simulink model "step6"  (Simulink 10.2)
settings: Solver=FixedStepAuto  StartTime=0.0  StopTime=3  FixedStep=T_step  RelTol=1e-3
values from neighbouring files (symbols this model uses):
  F = [Fx;Fy;Mz]    [Jacobi_T.m]    (also in PRBDM_CTC_task.m = M_tilda*v+C_tilda*dX+G_tilda; RRR_CTC_task.m = M_tilda*v+V_tilda*dX+G_tilda; RRR_jtraj.m = q0; step2.mat = 10)
  gama0 = Rparams4dyn(3)    [PRBDM_3R_Dynamic_Matrices_Lagrange.m]    (also in PRBDM_3R_Dynamics.m = in4dyn(12); PRBDM_3R_Dynamics00.m = in4dyn(12); PRBDM_3R_DynamicsPID.m = in4dyn(12); PRBDM_3R_parameters.m = 0.1)
  gama1 = x(7)    [Jacobi_T.m]    (also in PRBDM_3R_Dynamic_Matrices_Lagrange.m = Rparams4dyn(4); PRBDM_3R_Dynamics.m = in4dyn(13); PRBDM_3R_Dynamics00.m = in4dyn(13); PRBDM_3R_DynamicsPID.m = in4dyn(13))
  gama2 = x(8)    [Jacobi_T.m]    (also in PRBDM_3R_Dynamic_Matrices_Lagrange.m = Rparams4dyn(5); PRBDM_3R_Dynamics.m = in4dyn(14); PRBDM_3R_Dynamics00.m = in4dyn(14); PRBDM_3R_DynamicsPID.m = in4dyn(14))
  gama3 = x(9)    [Jacobi_T.m]    (also in PRBDM_3R_Dynamic_Matrices_Lagrange.m = Rparams4dyn(6); PRBDM_3R_Dynamics.m = in4dyn(15); PRBDM_3R_Dynamics00.m = in4dyn(15); PRBDM_3R_DynamicsPID.m = in4dyn(15))
  I = Rparams4dyn(10)    [PRBDM_3R_Dynamic_Matrices_Lagrange.m]    (also in PRBDM_3R_Dynamics.m = in4dyn(19); PRBDM_3R_Dynamics00.m = in4dyn(19); PRBDM_3R_DynamicsPID.m = in4dyn(19); PRBDM_3R_parameters.m = 1.8e-11)
  k1 = Rparams4dyn(7)    [PRBDM_3R_Dynamic_Matrices_Lagrange.m]    (also in PRBDM_3R_Dynamics.m = in4dyn(16); PRBDM_3R_Dynamics00.m = in4dyn(16); PRBDM_3R_DynamicsPID.m = in4dyn(16); PRBDM_3R_parameters.m = 0.290628)
  k2 = Rparams4dyn(8)    [PRBDM_3R_Dynamic_Matrices_Lagrange.m]    (also in PRBDM_3R_Dynamics.m = in4dyn(17); PRBDM_3R_Dynamics00.m = in4dyn(17); PRBDM_3R_DynamicsPID.m = in4dyn(17); PRBDM_3R_parameters.m = 0.247572)
  k3 = Rparams4dyn(9)    [PRBDM_3R_Dynamic_Matrices_Lagrange.m]    (also in PRBDM_3R_Dynamics.m = in4dyn(18); PRBDM_3R_Dynamics00.m = in4dyn(18); PRBDM_3R_DynamicsPID.m = in4dyn(18); PRBDM_3R_parameters.m = 0.213624)
  L = Rparams4dyn(2)    [PRBDM_3R_Dynamic_Matrices_Lagrange.m]    (also in PRBDM_3R_Dynamics.m = in4dyn(11); PRBDM_3R_Dynamics00.m = in4dyn(11); PRBDM_3R_DynamicsPID.m = in4dyn(11); PRBDM_3R_parameters.m = 0.3)
  L0 = z(7)    [Forward_kinematics.m]    (also in GeometricCalculation_simulink.m = Geoparams(4); PRBDM_3R_parameters.m = 0.03; PRBDM_3R_parameters.mat = 0.03; TrajectoryPlanning_simulink.m = X(8))
  L1 = z(8)    [Forward_kinematics.m]    (also in GeometricCalculation_simulink.m = Geoparams(5); Jacobi.m = x(4); PRBDM_3R_CTC.m = x(19); PRBDM_3R_Dynamic_Matrices_NewtonEular.m = robot_params(4))
  L2 = z(9)    [Forward_kinematics.m]    (also in GeometricCalculation_simulink.m = Geoparams(6); Jacobi.m = x(5); PRBDM_3R_CTC.m = x(20); PRBDM_3R_Dynamic_Matrices_NewtonEular.m = robot_params(5))
  L3 = z(10)    [Forward_kinematics.m]    (also in GeometricCalculation_simulink.m = Geoparams(7); Jacobi.m = x(6); PRBDM_3R_CTC.m = x(21); PRBDM_3R_Dynamic_Matrices_NewtonEular.m = robot_params(6))
  m = Rparams4dyn(1)    [PRBDM_3R_Dynamic_Matrices_Lagrange.m]    (also in PRBDM_3R_Dynamics.m = in4dyn(10); PRBDM_3R_Dynamics00.m = in4dyn(10); PRBDM_3R_DynamicsPID.m = in4dyn(10); PRBDM_3R_parameters.m = 1)
  Mz = x(6)    [Jacobi_T.m]    (also in step2.mat = 10; step2_trajectory.m = 10; step3.m = 10)
  phi_f = 1.0471975512    [step2.mat]    (also in step2_trajectory.m; step3.m)
  W = x(22)    [PRBDM_3R_CTC.m]    (also in PRBDM_3R_Dynamic_Matrices_NewtonEular.m = robot_params(7); PRBDM_3R_Dynamics.m = in4dyn(20); PRBDM_3R_Dynamics00.m = in4dyn(20); PRBDM_3R_DynamicsPID.m = in4dyn(20))
  x_f = 0.0536    [step2.mat]    (also in step2_trajectory.m; step3.m)
  y_f = 0.135    [step2.mat]    (also in step2_trajectory.m; step3.m)
settings Model: Creator=Master  LastModifiedBy=Master
settings DataIOCC: SaveFormat=Dataset  SignalLoggingSaveFormat=Dataset  ReturnWorkspaceOutputs=on
settings OptimizationCC: LifeSpan=auto
settings DebuggingCC: UnderspecifiedInitializationDetection=Simplified  MergeDetectMultiDrivingBlocksExec=error  FcnCallInpInsideContextMsg=error  SFUnexpectedBacktrackingDiag=error  SFNoUnconditionalDefaultTransitionDiag=error  SFExecutionAtInitializationDiag=warning  ArithmeticOperatorsInVariantConditions=error
settings HardwareCC: ProdBitPerPointer=64  ProdBitPerSizeT=64  ProdBitPerPtrDiffT=64  ProdLargestAtomicFloat=Float  ProdIntDivRoundTo=Zero  ProdEndianess=LittleEndian  ProdWordSize=64  ProdHWDeviceType=Intel->x86-64 (Windows64)
settings ModelReferenceCC: PropagateSignalLabelsOutOfModel=on
settings SFSimCC: SimUseLocalCustomCode=on  CustomCodeUndefinedFunction=FilterOut
settings RTWCC: RTWUseLocalCustomCode=on
settings CodeAppCC: StateflowObjectComments=off
settings GRTTargetCC: TargetLangStandard=C99 (ISO)  CombineOutputUpdateFcns=on  GRTInterface=off
settings ConfigComp: CovMetricSettings=dwe  CovSaveCumulativeToWorkspaceVar=off  CovSaveSingleToWorkspaceVar=off  CovExternalEMLEnable=on

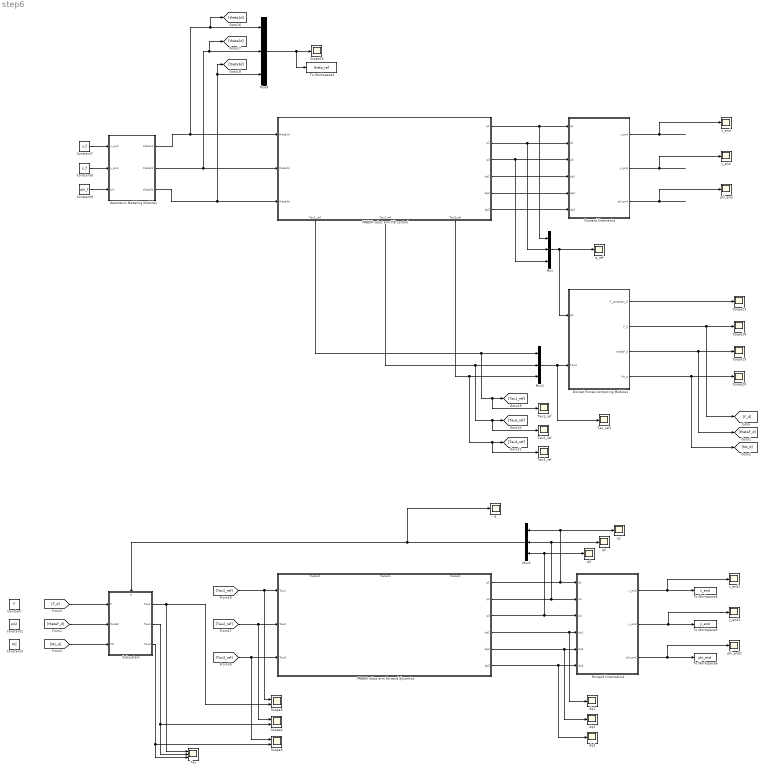
== system step6 ==
  Constant : Constant  Value=F
  Constant1 : Constant  Value=pi/2
  Constant3 : Constant  Value=Mz
  Constant7 : Constant  Value=x_f
  Constant8 : Constant  Value=y_f
  Constant9 : Constant  Value=phi_f
  Disired Forces Computing Module1 : Subsystem
  Forward kinematics : Subsystem
  Forward kinematics1 : Subsystem
  Geometric Modeling Module1 : Subsystem
  Mux{,1..2,9} (4 alike) : Mux  Inputs=3
  PRBDM robot arm Forward dynamics : Subsystem
      settings: PortSchema="{\"entries\":[{\"content\":{\"sides\":[{\"content\":{\"connectorIds\":[\"In1\",\"In2\",\"In3\"]},\"type\":\"ConnectorPlacement.EquallySpacedRectSide\",\"uuid\":\"1f88892b-0bd0-49de-aca9-2c32e7693572\"},{\"content\":{\"connectorIds\":[\"Out1\",\"Out2\",\"Out3\",\"Out4\",\"Out5\",\"Out6\"],\"side\":\"RIGHT\"},\"type\":\"ConnectorPlacement.EquallySpacedRectSide\",\"uuid\":\"b703a21d-fa56-4217-8064-1c2098ab3c38\"},{\"content\":{\"connectorIds\":[\"In4\",\"In5\",\"In6\"],\"side\":\"TOP\"},\"type\":\"ConnectorPlacement.EquallySpacedRectSide\",\"uuid\":\"2526ef97-18a1-4ac3-963d-0ba7d1a2d319\"},{\"content\":{\"connectorIds\":[],\"side\":\"BOTTOM\"},\"type\":\"ConnectorPlacement.EquallySpacedRectSide\",\"uuid\":\"f33fbcfd-8e0b-408f-a669-776188a4cff3\"},{\"content\":{\"connectorIds\":[],\"side\":\"HIDDEN\"},\"type\":\"ConnectorPlacement.EquallySpacedRectSide\",\"uuid\":\"8c9044ff-40c0-4995-b32e-bf50be4b71db\"}]},\"type\":\"ConnectorPlacement.EquallySpacedConnector\",\"uuid\":\"32b5ad01-d59a-45fa-aad8-e0a4c9d304fb\"}],\"packageUris\":[\"http://schema.mathworks.com/mf0/Connector/R2020b\"],\"version\":\"1.0\"}"
      mask Display: image(imread('RRR.png'))
  PRBDM robot arm PID control : Subsystem
      settings: PortSchema="{\"entries\":[{\"content\":{\"sides\":[{\"content\":{\"connectorIds\":[\"In1\",\"In2\",\"In3\"]},\"type\":\"ConnectorPlacement.EquallySpacedRectSide\",\"uuid\":\"1f88892b-0bd0-49de-aca9-2c32e7693572\"},{\"content\":{\"connectorIds\":[\"Out1\",\"Out2\",\"Out3\",\"Out4\",\"Out5\",\"Out6\"],\"side\":\"RIGHT\"},\"type\":\"ConnectorPlacement.EquallySpacedRectSide\",\"uuid\":\"b703a21d-fa56-4217-8064-1c2098ab3c38\"},{\"content\":{\"connectorIds\":[],\"side\":\"TOP\"},\"type\":\"ConnectorPlacement.EquallySpacedRectSide\",\"uuid\":\"2526ef97-18a1-4ac3-963d-0ba7d1a2d319\"},{\"content\":{\"connectorIds\":[\"Out7\",\"Out8\",\"Out9\"],\"side\":\"BOTTOM\"},\"type\":\"ConnectorPlacement.EquallySpacedRectSide\",\"uuid\":\"f33fbcfd-8e0b-408f-a669-776188a4cff3\"},{\"content\":{\"connectorIds\":[],\"side\":\"HIDDEN\"},\"type\":\"ConnectorPlacement.EquallySpacedRectSide\",\"uuid\":\"8c9044ff-40c0-4995-b32e-bf50be4b71db\"}]},\"type\":\"ConnectorPlacement.EquallySpacedConnector\",\"uuid\":\"32b5ad01-d59a-45fa-aad8-e0a4c9d304fb\"}],\"packageUris\":[\"http://schema.mathworks.com/mf0/Connector/R2020b\"],\"version\":\"1.0\"}"
      mask Display: image(imread('RRR.png'))
  Scope{16,18..20,23} (5 alike) : Scope
  Scope2 : Scope  NumInputPorts=2
  Scope3 : Scope  NumInputPorts=2
  Scope5 : Scope  NumInputPorts=2
  Subsystem : Subsystem
      settings: PortSchema="{\"entries\":[{\"content\":{\"sides\":[{\"content\":{\"connectorIds\":[\"In1\",\"In2\",\"In3\"]},\"type\":\"ConnectorPlacement.EquallySpacedRectSide\",\"uuid\":\"03e3fa68-98df-40a7-88fb-f274e89646de\"},{\"content\":{\"connectorIds\":[\"Out1\",\"Out2\",\"Out3\"],\"side\":\"RIGHT\"},\"type\":\"ConnectorPlacement.EquallySpacedRectSide\",\"uuid\":\"1a7c6e69-d785-4f03-b0d8-74a38f8f42a1\"},{\"content\":{\"connectorIds\":[\"In4\"],\"side\":\"TOP\"},\"type\":\"ConnectorPlacement.EquallySpacedRectSide\",\"uuid\":\"61c135cb-8cc5-493d-9c37-8230cda997e1\"},{\"content\":{\"connectorIds\":[],\"side\":\"HIDDEN\"},\"type\":\"ConnectorPlacement.EquallySpacedRectSide\",\"uuid\":\"5d99950e-feb6-474c-993a-cad470b06503\"}]},\"type\":\"ConnectorPlacement.EquallySpacedConnector\",\"uuid\":\"5533c5e9-db4a-4e3a-8115-8d67f8979e0c\"}],\"packageUris\":[\"http://schema.mathworks.com/mf0/Connector/R2020b\"],\"version\":\"1.0\"}"
  Tau : Scope  NumInputPorts=3
  Tau1_ref : Scope
  Tau2_ref : Scope
  Tau3_ref : Scope
  Tau_ref1 : Scope
  To Workspace3 : ToWorkspace  VariableName=theta_ref  SaveFormat=Timeseries  SampleTime=-1
  To Workspace4 : ToWorkspace  VariableName=x_end  SampleTime=-1
  To Workspace5 : ToWorkspace  VariableName=y_end  SampleTime=-1
  To Workspace6 : ToWorkspace  VariableName=phi_end  SampleTime=-1
  dq1 : Scope
  dq2 : Scope
  dq3 : Scope
  phi_end : Scope
  phi_end1 : Scope
  q{,1..3} (4 alike) : Scope
  q_ref : Scope
  x_end : Scope
  x_end1 : Scope
  y_end : Scope
  y_end1 : Scope
  wires:
  Mux9/1 -> To Workspace3/1, Scope16/1
  Geometric Modeling Module1/3(theta3d) -> [theta3d], Mux9/3, PRBDM robot arm PID control/3(theta3d)
  Constant9/1 -> Geometric Modeling Module1/3(phi)
  Constant7/1 -> Geometric Modeling Module1/1(x_end)
  Constant8/1 -> Geometric Modeling Module1/2(y_end)
  Geometric Modeling Module1/1(theta1d) -> PRBDM robot arm PID control/1(theta1d), [theta1d], Mux9/1
  Geometric Modeling Module1/2(theta2d) -> PRBDM robot arm PID control/2(theta2d), [theta2d], Mux9/2
  Mux/1 -> q_ref/1, Disired Forces Computing Module1/1(qd)
  PRBDM robot arm PID control/5(dq2) -> Forward kinematics/5(dq2)
  PRBDM robot arm PID control/1(q1) -> Mux/1, Forward kinematics/1(q1)
  PRBDM robot arm PID control/6(dq3) -> Forward kinematics/6(dq3)
  PRBDM robot arm PID control/4(dq1) -> Forward kinematics/4(dq1)
  Forward kinematics/1(x_end) -> x_end/1
  PRBDM robot arm PID control/2(q2) -> Forward kinematics/2(q2), Mux/2
  Forward kinematics/3(phi_end) -> phi_end/1
  Forward kinematics/2(y_end) -> y_end/1
  PRBDM robot arm PID control/3(q3) -> Forward kinematics/3(q3), Mux/3
  Disired Forces Computing Module1/4(Mz_d) -> [Mz_d], Scope20/1
  Disired Forces Computing Module1/3(thetaF_d) -> [thetaF_d], Scope19/1
  Disired Forces Computing Module1/2(F_d) -> [F_d], Scope18/1
  Disired Forces Computing Module1/1(F_cartesian_d) -> Scope23/1
  PRBDM robot arm PID control/8(Tau2_ref) -> Tau2_ref/1, [Tau2_ref], Mux1/2
  PRBDM robot arm PID control/7(Tau1_ref) -> Tau1_ref/1, [Tau1_ref], Mux1/1
  Mux1/1 -> Tau_ref1/1, Disired Forces Computing Module1/2(Taud)
  PRBDM robot arm PID control/9(Tau3_ref) -> Tau3_ref/1, [Tau3_ref], Mux1/3
  Forward kinematics1/2(y_end) -> y_end1/1, To Workspace5/1
  PRBDM robot arm Forward dynamics/2(q2) -> q2/1, Mux2/2, Forward kinematics1/2(q2)
  PRBDM robot arm Forward dynamics/3(q3) -> q3/1, Mux2/3, Forward kinematics1/3(q3)
  Forward kinematics1/1(x_end) -> To Workspace4/1, x_end1/1
  PRBDM robot arm Forward dynamics/4(dq1) -> dq1/1, Forward kinematics1/4(dq1)
  PRBDM robot arm Forward dynamics/6(dq3) -> dq3/1, Forward kinematics1/6(dq3)
  PRBDM robot arm Forward dynamics/5(dq2) -> dq2/1, Forward kinematics1/5(dq2)
  PRBDM robot arm Forward dynamics/1(q1) -> Mux2/1, q1/1, Forward kinematics1/1(q1)
  Mux2/1 -> Subsystem/4(q), q/1
  Forward kinematics1/3(phi_end) -> phi_end1/1, To Workspace6/1
  [Mz_d] -> Subsystem/3(Mz)
  [thetaF_d] -> Subsystem/2(thetaF)
  [F_d] -> Subsystem/1(F)
  [Tau1_ref] -> Scope5/1, PRBDM robot arm Forward dynamics/1(Tau1)
  [Tau2_ref] -> Scope2/1, PRBDM robot arm Forward dynamics/2(Tau2)
  [Tau3_ref] -> Scope3/1, PRBDM robot arm Forward dynamics/3(Tau3)
  Subsystem/1(Tau1) -> Tau/1, Scope5/2
  Subsystem/2(Tau2) -> Scope2/2, Tau/2
  Subsystem/3(Tau3) -> Scope3/2, Tau/3

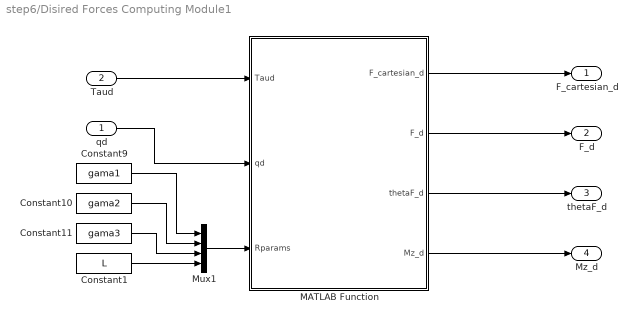
== system step6/Disired Forces Computing Module1 ==
  qd : Inport
  Taud : Inport  Port=2
  Constant1 : Constant  Value=L
  Constant10 : Constant  Value=gama2
  Constant11 : Constant  Value=gama3
  Constant9 : Constant  Value=gama1
  MATLAB Function : MATLAB Function  TreatAsAtomicUnit=on
  Mux1 : Mux
  F_cartesian_d : Outport
  F_d : Outport  Port=2
  thetaF_d : Outport  Port=3
  Mz_d : Outport  Port=4
  wires:
  MATLAB Function/1(F_cartesian_d) -> F_cartesian_d/1
  Mux1/1 -> MATLAB Function/3(Rparams)
  Constant9/1 -> Mux1/1
  Constant10/1 -> Mux1/2
  Constant11/1 -> Mux1/3
  Taud/1 -> MATLAB Function/1(Taud)
  qd/1 -> MATLAB Function/2(qd)
  Constant1/1 -> Mux1/4
  MATLAB Function/2(F_d) -> F_d/1
  MATLAB Function/3(thetaF_d) -> thetaF_d/1
  MATLAB Function/4(Mz_d) -> Mz_d/1

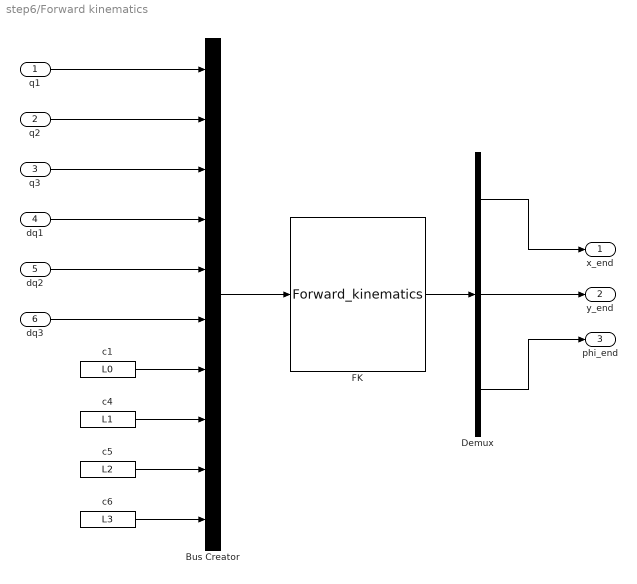
== system step6/Forward kinematics ==
  q1 : Inport
  q2 : Inport  Port=2
  q3 : Inport  Port=3
  dq1 : Inport  Port=4
  dq2 : Inport  Port=5
  dq3 : Inport  Port=6
  Bus Creator : BusCreator  Inputs=10
  Demux : Demux  Outputs=3
  FK : MATLABFcn  MATLABFcn=Forward_kinematics  OutputDimensions=3
  c1 : Constant  Value=L0
  c4 : Constant  Value=L1
  c5 : Constant  Value=L2
  c6 : Constant  Value=L3
  x_end : Outport
  y_end : Outport  Port=2
  phi_end : Outport  Port=3
  wires:
  c6/1 -> Bus Creator/10
  Demux/1 -> x_end/1
  c4/1 -> Bus Creator/8
  q2/1 -> Bus Creator/2
  q1/1 -> Bus Creator/1
  q3/1 -> Bus Creator/3
  Bus Creator/1 -> FK/1
  dq2/1 -> Bus Creator/5
  Demux/2 -> y_end/1
  FK/1 -> Demux/1
  dq1/1 -> Bus Creator/4
  Demux/3 -> phi_end/1
  dq3/1 -> Bus Creator/6
  c5/1 -> Bus Creator/9
  c1/1 -> Bus Creator/7

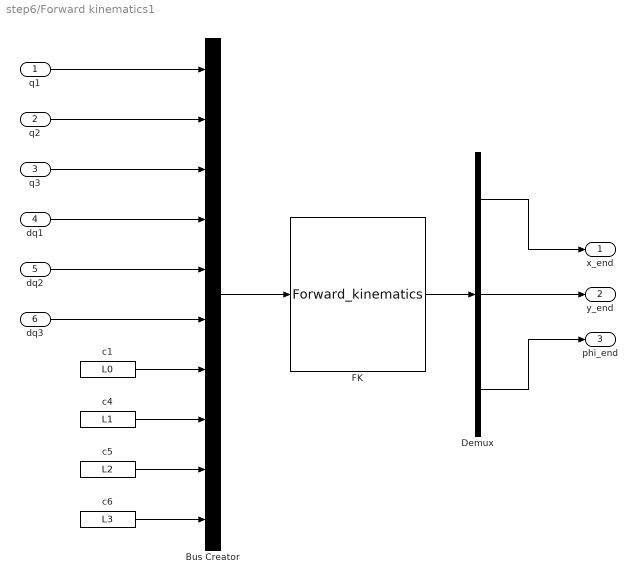
== system step6/Forward kinematics1 ==
  q1 : Inport
  q2 : Inport  Port=2
  q3 : Inport  Port=3
  dq1 : Inport  Port=4
  dq2 : Inport  Port=5
  dq3 : Inport  Port=6
  Bus Creator : BusCreator  Inputs=10
  Demux : Demux  Outputs=3
  FK : MATLABFcn  MATLABFcn=Forward_kinematics  OutputDimensions=3
  c1 : Constant  Value=L0
  c4 : Constant  Value=L1
  c5 : Constant  Value=L2
  c6 : Constant  Value=L3
  x_end : Outport
  y_end : Outport  Port=2
  phi_end : Outport  Port=3
  wires:
  c6/1 -> Bus Creator/10
  Demux/1 -> x_end/1
  c4/1 -> Bus Creator/8
  q2/1 -> Bus Creator/2
  q1/1 -> Bus Creator/1
  q3/1 -> Bus Creator/3
  Bus Creator/1 -> FK/1
  dq2/1 -> Bus Creator/5
  Demux/2 -> y_end/1
  FK/1 -> Demux/1
  dq1/1 -> Bus Creator/4
  Demux/3 -> phi_end/1
  dq3/1 -> Bus Creator/6
  c5/1 -> Bus Creator/9
  c1/1 -> Bus Creator/7

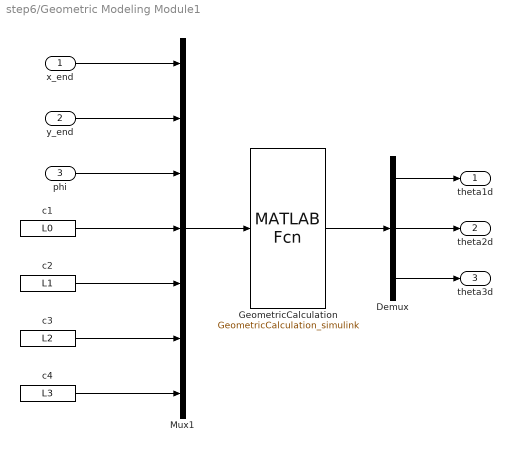
== system step6/Geometric Modeling Module1 ==
  x_end : Inport
  y_end : Inport  Port=2
  phi : Inport  Port=3
  Demux : Demux  Outputs=3
  GeometricCalculation : MATLABFcn  MATLABFcn=GeometricCalculation_simulink
  Mux1 : Mux  Inputs=7
  c1 : Constant  Value=L0
  c2 : Constant  Value=L1
  c3 : Constant  Value=L2
  c4 : Constant  Value=L3
  theta1d : Outport
  theta2d : Outport  Port=2
  theta3d : Outport  Port=3
  wires:
  Mux1/1 -> GeometricCalculation/1
  y_end/1 -> Mux1/2
  x_end/1 -> Mux1/1
  phi/1 -> Mux1/3
  c1/1 -> Mux1/4
  c3/1 -> Mux1/6
  c2/1 -> Mux1/5
  GeometricCalculation/1 -> Demux/1
  Demux/2 -> theta2d/1
  Demux/1 -> theta1d/1
  Demux/3 -> theta3d/1
  c4/1 -> Mux1/7

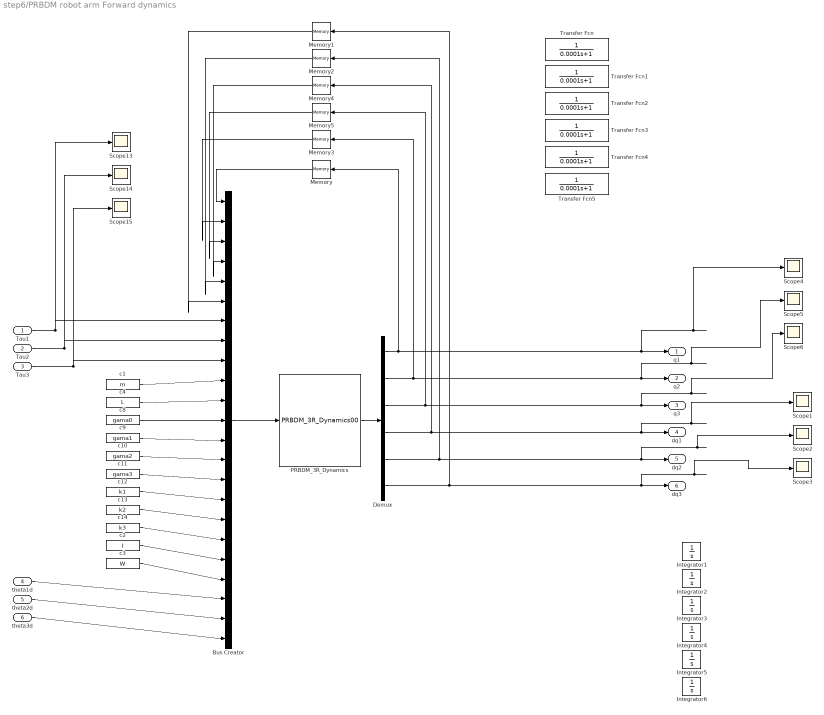
== system step6/PRBDM robot arm Forward dynamics ==
  Tau1 : Inport
  Tau2 : Inport  Port=2
  Tau3 : Inport  Port=3
  theta1d : Inport  Port=4
  theta2d : Inport  Port=5
  theta3d : Inport  Port=6
  Bus Creator : BusCreator  Inputs=23
  Demux : Demux  Outputs=6
  Integrator{1..6} (6 alike) : Integrator  UpperSaturationLimit=1e6  LowerSaturationLimit=-1e6
  Memory{,1..5} (6 alike) : Memory
  PRBDM_3R_Dynamics : MATLABFcn  MATLABFcn=PRBDM_3R_Dynamics00  OutputDimensions=6
  Scope{1..6,13..15} (9 alike) : Scope
  Transfer Fcn{,1..5} (6 alike) : TransferFcn  Denominator=[0.0001 1]
  c1 : Constant  Value=m
  c10 : Constant  Value=gama2
  c11 : Constant  Value=gama3
  c12 : Constant  Value=k1
  c13 : Constant  Value=k2
  c14 : Constant  Value=k3
  c2 : Constant  Value=I
  c3 : Constant  Value=W
  c4 : Constant  Value=L
  c8 : Constant  Value=gama0
  c9 : Constant  Value=gama1
  q1 : Outport
  q2 : Outport  Port=2
  q3 : Outport  Port=3
  dq1 : Outport  Port=4
  dq2 : Outport  Port=5
  dq3 : Outport  Port=6
  wires:
  theta3d/1 -> Bus Creator/23
  theta2d/1 -> Bus Creator/22
  c11/1 -> Bus Creator/15
  c3/1 -> Bus Creator/20
  c14/1 -> Bus Creator/18
  c2/1 -> Bus Creator/19
  c1/1 -> Bus Creator/10
  c8/1 -> Bus Creator/12
  Bus Creator/1 -> PRBDM_3R_Dynamics/1
  Tau1/1 -> Scope13/1, Bus Creator/7
  PRBDM_3R_Dynamics/1 -> Demux/1
  c4/1 -> Bus Creator/11
  c10/1 -> Bus Creator/14
  c9/1 -> Bus Creator/13
  c13/1 -> Bus Creator/17
  Tau3/1 -> Scope15/1, Bus Creator/9
  c12/1 -> Bus Creator/16
  theta1d/1 -> Bus Creator/21
  Tau2/1 -> Scope14/1, Bus Creator/8
  Demux/1 -> Memory/1, q1/1, Scope4/1
  Demux/2 -> Memory3/1, q2/1, Scope5/1
  Demux/3 -> Memory5/1, q3/1, Scope6/1
  Demux/4 -> Memory4/1, dq1/1, Scope1/1
  Demux/5 -> Memory2/1, dq2/1, Scope2/1
  Demux/6 -> Memory1/1, dq3/1, Scope3/1
  Memory/1 -> Bus Creator/1
  Memory3/1 -> Bus Creator/2
  Memory5/1 -> Bus Creator/3
  Memory4/1 -> Bus Creator/4
  Memory2/1 -> Bus Creator/5
  Memory1/1 -> Bus Creator/6

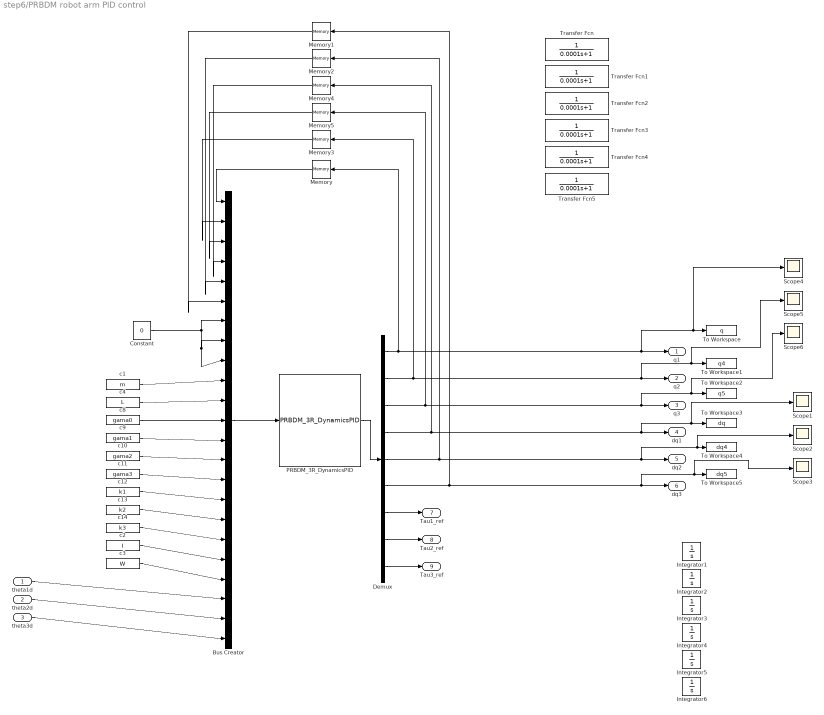
== system step6/PRBDM robot arm PID control ==
  theta1d : Inport
  theta2d : Inport  Port=2
  theta3d : Inport  Port=3
  Bus Creator : BusCreator  Inputs=23
  Constant : Constant  Value=0
  Demux : Demux  Outputs=9
  Integrator{1..6} (6 alike) : Integrator  UpperSaturationLimit=1e6  LowerSaturationLimit=-1e6
  Memory{,1..5} (6 alike) : Memory
  PRBDM_3R_DynamicsPID : MATLABFcn  MATLABFcn=PRBDM_3R_DynamicsPID  OutputDimensions=9
  Scope{1..6} (6 alike) : Scope
  To Workspace : ToWorkspace  VariableName=q  SampleTime=-1
  To Workspace1 : ToWorkspace  VariableName=q4  SampleTime=-1
  To Workspace2 : ToWorkspace  VariableName=q5  SampleTime=-1
  To Workspace3 : ToWorkspace  VariableName=dq  SampleTime=-1
  To Workspace4 : ToWorkspace  VariableName=dq4  SampleTime=-1
  To Workspace5 : ToWorkspace  VariableName=dq5  SampleTime=-1
  Transfer Fcn{,1..5} (6 alike) : TransferFcn  Denominator=[0.0001 1]
  c1 : Constant  Value=m
  c10 : Constant  Value=gama2
  c11 : Constant  Value=gama3
  c12 : Constant  Value=k1
  c13 : Constant  Value=k2
  c14 : Constant  Value=k3
  c2 : Constant  Value=I
  c3 : Constant  Value=W
  c4 : Constant  Value=L
  c8 : Constant  Value=gama0
  c9 : Constant  Value=gama1
  q1 : Outport
  q2 : Outport  Port=2
  q3 : Outport  Port=3
  dq1 : Outport  Port=4
  dq2 : Outport  Port=5
  dq3 : Outport  Port=6
  Tau1_ref : Outport  Port=7
  Tau2_ref : Outport  Port=8
  Tau3_ref : Outport  Port=9
  wires:
  theta3d/1 -> Bus Creator/23
  theta2d/1 -> Bus Creator/22
  c11/1 -> Bus Creator/15
  c3/1 -> Bus Creator/20
  c14/1 -> Bus Creator/18
  c2/1 -> Bus Creator/19
  c1/1 -> Bus Creator/10
  c8/1 -> Bus Creator/12
  Bus Creator/1 -> PRBDM_3R_DynamicsPID/1
  PRBDM_3R_DynamicsPID/1 -> Demux/1
  c4/1 -> Bus Creator/11
  c10/1 -> Bus Creator/14
  c9/1 -> Bus Creator/13
  c13/1 -> Bus Creator/17
  c12/1 -> Bus Creator/16
  theta1d/1 -> Bus Creator/21
  Demux/1 -> Memory/1, q1/1, Scope4/1, To Workspace/1
  Demux/2 -> Memory3/1, q2/1, Scope5/1, To Workspace1/1
  Demux/3 -> Memory5/1, q3/1, Scope6/1, To Workspace2/1
  Demux/4 -> Memory4/1, dq1/1, Scope1/1, To Workspace3/1
  Demux/5 -> Memory2/1, dq2/1, Scope2/1, To Workspace4/1
  Demux/6 -> Memory1/1, dq3/1, Scope3/1, To Workspace5/1
  Memory/1 -> Bus Creator/1
  Memory3/1 -> Bus Creator/2
  Memory5/1 -> Bus Creator/3
  Memory4/1 -> Bus Creator/4
  Memory2/1 -> Bus Creator/5
  Memory1/1 -> Bus Creator/6
  Demux/7 -> Tau1_ref/1
  Demux/8 -> Tau2_ref/1
  Demux/9 -> Tau3_ref/1
  Constant/1 -> Bus Creator/9, Bus Creator/8, Bus Creator/7

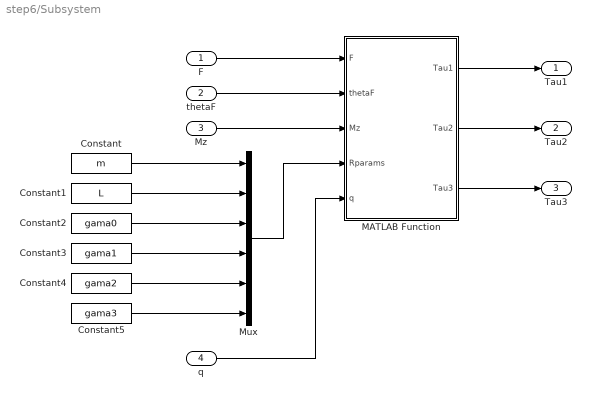
== system step6/Subsystem ==
  F : Inport
  thetaF : Inport  Port=2
  Mz : Inport  Port=3
  q : Inport  Port=4
  Constant : Constant  Value=m
  Constant1 : Constant  Value=L
  Constant2 : Constant  Value=gama0
  Constant3 : Constant  Value=gama1
  Constant4 : Constant  Value=gama2
  Constant5 : Constant  Value=gama3
  MATLAB Function : MATLAB Function  TreatAsAtomicUnit=on
  Mux : Mux  Inputs=6
  Tau1 : Outport
  Tau2 : Outport  Port=2
  Tau3 : Outport  Port=3
  wires:
  thetaF/1 -> MATLAB Function/2(thetaF)
  F/1 -> MATLAB Function/1(F)
  Mz/1 -> MATLAB Function/3(Mz)
  MATLAB Function/1(Tau1) -> Tau1/1
  Constant/1 -> Mux/1
  Constant1/1 -> Mux/2
  Constant2/1 -> Mux/3
  Constant3/1 -> Mux/4
  Constant4/1 -> Mux/5
  Constant5/1 -> Mux/6
  Mux/1 -> MATLAB Function/4(Rparams)
  MATLAB Function/2(Tau2) -> Tau2/1
  MATLAB Function/3(Tau3) -> Tau3/1
  q/1 -> MATLAB Function/5(q)

== matlab function Subsystem/MATLAB Function ==
  data: F input double; thetaF input double; Tau1 output double; Mz input double; Rparams input double; q input double; Tau2 output double; Tau3 output double
function [Tau1,Tau2, Tau3] = fcn(F, thetaF, Mz, Rparams, q)

m = Rparams(1);
L = Rparams(2);
gama0 = Rparams(3);
gama1 = Rparams(4);
gama2 = Rparams(5);
gama3 = Rparams(6);


FxL = F*L*cos(thetaF);
FyL = F*L*sin(thetaF);
F_cartesian = [FxL; FyL; Mz];

Rparams4J = zeros(4);
Rparams4J(1) = gama1;
Rparams4J(2) = gama2;
Rparams4J(3) = gama3;
Rparams4J(4) = L;
J = PRBDM_3R_Jacobi(q,Rparams4J);

J_T = transpose(J);

Tau = J_T*F_cartesian;
Tau1 = Tau(1);
Tau2 = Tau(2);
Tau3 = Tau(3);

== matlab function Disired Forces Computing Module1/MATLAB Function ==
  data: Taud input double; F_cartesian_d output double; qd input double; Rparams input double; F_d output double; thetaF_d output double; Mz_d output double
function [F_cartesian_d, F_d, thetaF_d, Mz_d] = DesiredForcesComputing(Taud,qd,Rparams)

% Rparams4J;
gama1 = Rparams(1);
gama2 = Rparams(2);
gama3 = Rparams(3);
L = Rparams(4);

Rparams4J = [gama1 gama2 gama3];

J = PRBDM_3R_Jacobi(qd,Rparams4J);
J_T = transpose(J);


% F_cartesian = inv(J_T) * Taud;
F_cartesian_d = J_T \ Taud;

FxL = F_cartesian_d(1);
FyL = F_cartesian_d(2);
Mz = F_cartesian_d(3);

thetaF_d = atan2(FyL,FxL);
F_d = FxL/L/cos(thetaF_d);
Mz_d = Mz;
